simulink model "TA_TKO"  (R2021a)
settings: Solver=VariableStepAuto  StartTime=0.0  StopTime=10.0  RelTol=1e-3
values from neighbouring files (symbols this model uses):
  den = [La * J, (La * B + Ra * J), (Ra * B + Kb * K)]    [TA_TKO_FUNGSI ALIH.m]    (also in TA_TKO_FUNGSIALIH.m)
  num = K    (= 0.015)    [TA_TKO_FUNGSI ALIH.m]    (also in TA_TKO_FUNGSIALIH.m)
settings Model: Creator=Annas  LastModifiedBy=Annas

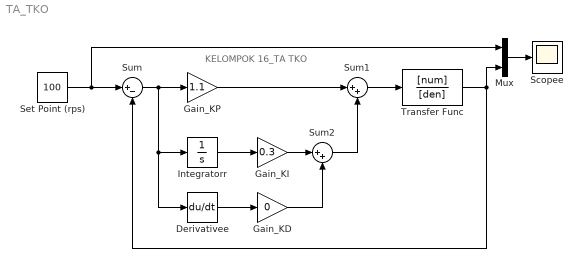
== system TA_TKO ==
  note: KELOMPOK 16_TA TKO
  Derivativee : Derivative
  Gain_KD : Gain  Gain=0
  Gain_KI : Gain  Gain=0.3
  Gain_KP : Gain  Gain=1.1
  Integratorr : Integrator
  Mux : Mux  Inputs=2
  Scopee : Scope
  Set Point (rps) : Constant  Value=100
  Sum : Sum  Inputs=|+-
  Sum1 : Sum  Inputs=|++
  Sum2 : Sum  Inputs=|++
  Transfer Func : TransferFcn  Numerator=[num]  Denominator=[den]
  wires:
  Sum1/1 -> Transfer Func/1
  Set Point (rps)/1 -> Mux/1, Sum/1
  Sum/1 -> Derivativee/1, Integratorr/1, Gain_KP/1
  Gain_KP/1 -> Sum1/1
  Integratorr/1 -> Gain_KI/1
  Derivativee/1 -> Gain_KD/1
  Transfer Func/1 -> Sum/2, Mux/2
  Mux/1 -> Scopee/1
  Gain_KI/1 -> Sum2/1
  Gain_KD/1 -> Sum2/2
  Sum2/1 -> Sum1/2
